simulink model "P_controller"  (R2023a)
settings: Solver=VariableStepAuto  StartTime=0.0  StopTime=100  RelTol=1e-3
values from neighbouring files (symbols this model uses):
  dem = [taux 1]    [servo_simulation.m]
settings Model: Creator=IDEAL SOFT  LastModifiedBy=IDEAL SOFT

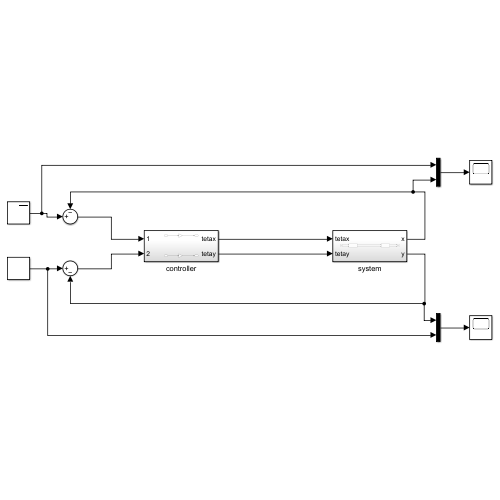
[thumbnail: Simulink's stored preview of the top-level diagram]
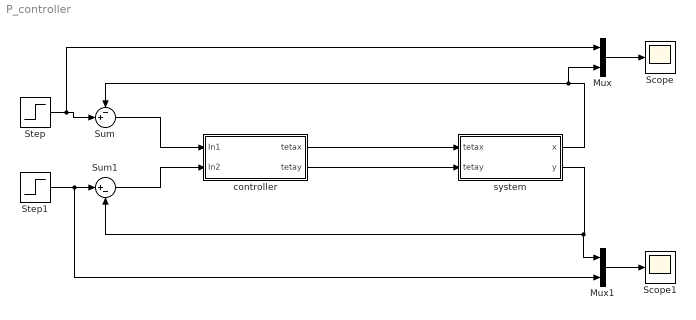
== system P_controller ==
  Mux : Mux  Inputs=2
  Mux1 : Mux  Inputs=2
  Scope : Scope
  Scope1 : Scope
  Step : Step  After=0  SampleTime=0
  Step1 : Step  After=30  SampleTime=0
  Sum : Sum  Inputs=-+|
  Sum1 : Sum  Inputs=|+-
  controller : Subsystem
  system : Subsystem
  wires:
  controller/1(tetax) -> system/1(tetax)
  controller/2(tetay) -> system/2(tetay)
  system/1(x) -> Mux/2, Sum/1
  system/2(y) -> Mux1/1, Sum1/2
  Sum/1 -> controller/1(In1)
  Sum1/1 -> controller/2(In2)
  Step/1 -> Mux/1, Sum/2
  Step1/1 -> Mux1/2, Sum1/1
  Mux1/1 -> Scope1/1
  Mux/1 -> Scope/1

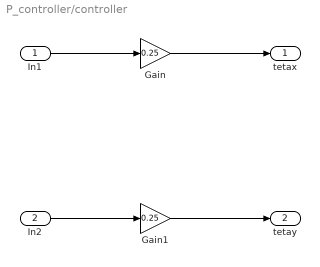
== system P_controller/controller ==
  In1 : Inport
  In2 : Inport  Port=2
  Gain : Gain  Gain=0.25
  Gain1 : Gain  Gain=0.25
  tetax : Outport
  tetay : Outport  Port=2
  wires:
  In1/1 -> Gain/1
  Gain/1 -> tetax/1
  In2/1 -> Gain1/1
  Gain1/1 -> tetay/1

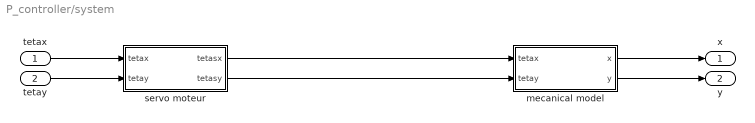
== system P_controller/system ==
  tetax : Inport
  tetay : Inport  Port=2
  mecanical model : Subsystem
  servo moteur : Subsystem
  x : Outport
  y : Outport  Port=2
  wires:
  servo moteur/2(tetasy) -> mecanical model/2(tetay)
  servo moteur/1(tetasx) -> mecanical model/1(tetax)
  mecanical model/2(y) -> y/1
  mecanical model/1(x) -> x/1
  tetax/1 -> servo moteur/1(tetax)
  tetay/1 -> servo moteur/2(tetay)

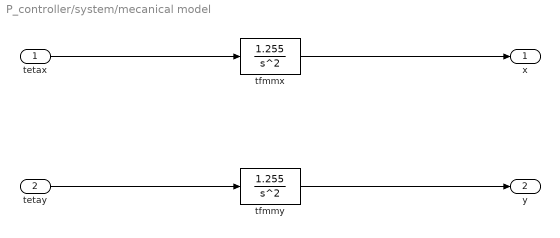
== system P_controller/system/mecanical model ==
  tetax : Inport
  tetay : Inport  Port=2
  tfmmx : TransferFcn  Numerator=1.255  Denominator=[1 0 0]
  tfmmy : TransferFcn  Numerator=1.255  Denominator=[1 0 0]
  x : Outport
  y : Outport  Port=2
  wires:
  tetax/1 -> tfmmx/1
  tfmmx/1 -> x/1
  tetay/1 -> tfmmy/1
  tfmmy/1 -> y/1

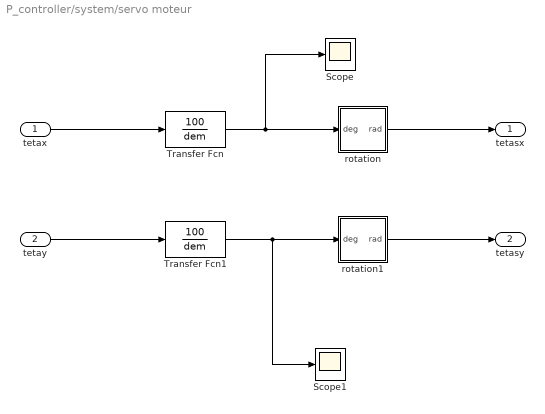
== system P_controller/system/servo moteur ==
  tetax : Inport
  tetay : Inport  Port=2
  Scope : Scope
  Scope1 : Scope
  Transfer Fcn : TransferFcn  Numerator=100  Denominator=dem
  Transfer Fcn1 : TransferFcn  Numerator=100  Denominator=dem
  rotation : Subsystem
  rotation1 : Subsystem
  tetasx : Outport
  tetasy : Outport  Port=2
  wires:
  tetax/1 -> Transfer Fcn/1
  tetay/1 -> Transfer Fcn1/1
  Transfer Fcn/1 -> Scope/1, rotation/1(deg)
  rotation/1(rad) -> tetasx/1
  Transfer Fcn1/1 -> Scope1/1, rotation1/1(deg)
  rotation1/1(rad) -> tetasy/1

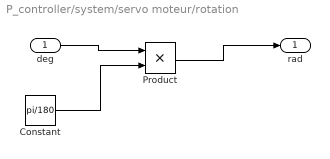
== system P_controller/system/servo moteur/rotation ==
  deg : Inport
  Constant : Constant  Value=pi/180
  Product : Product
  rad : Outport
  wires:
  deg/1 -> Product/1
  Product/1 -> rad/1
  Constant/1 -> Product/2

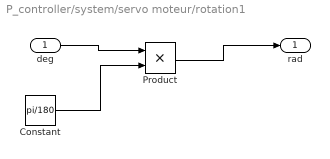
== system P_controller/system/servo moteur/rotation1 ==
  deg : Inport
  Constant : Constant  Value=pi/180
  Product : Product
  rad : Outport
  wires:
  deg/1 -> Product/1
  Product/1 -> rad/1
  Constant/1 -> Product/2
